simulink model "Guidance"  (R2026a)
settings: Solver=VariableStepAuto
undefined symbols (not defined in the file): ts_uav, waypoints
settings Model: DataDictionary=QuadData.sldd  ModifiedByFormat=The MathWorks, Inc.  Creator=The MathWorks, Inc.  LastModifiedBy=The MathWorks, Inc.

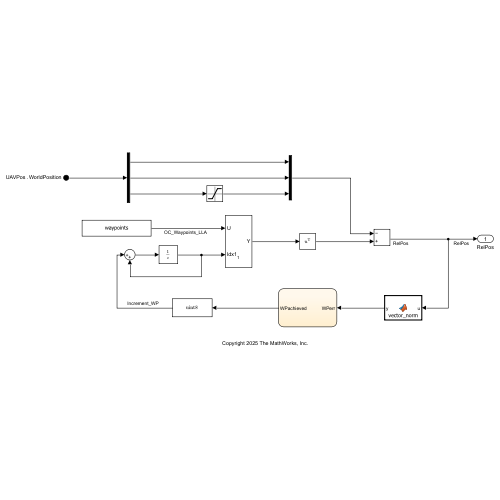
[thumbnail: Simulink's stored preview of the top-level diagram]
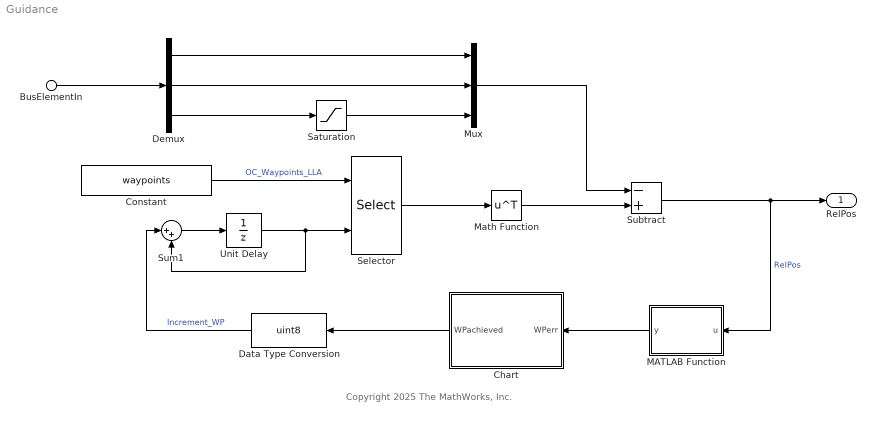
== system Guidance ==
  note: Copyright 2025 The MathWorks, Inc.
  BusElementIn : Inport  PortName=UAVPos  Element=WorldPosition
  Chart : Stateflow chart  TreatAsAtomicUnit=on
  Constant : Constant  Value=waypoints  SampleTime=ts_uav
  Data Type Conversion : DataTypeConversion  OutDataTypeStr=uint8  SaturateOnIntegerOverflow=off  RndMeth=Floor
  Demux : Demux  Outputs=3
  MATLAB Function : MATLAB Function  TreatAsAtomicUnit=on
  Math Function : Math  Operator=transpose
  Mux : Mux  Inputs=3
  Saturation : Saturate  UpperLimit=0.0001  LowerLimit=-inf
  Selector : Selector  NumberOfDimensions=2  InputPortWidth=3  IndexOptions=Starting index (port),Select all  Indices=[1 3],1  OutputSizes=1,1
  Subtract : Sum  Inputs=-+
  Sum1 : Sum  Inputs=|++
  Unit Delay : UnitDelay  InitialCondition=1  SampleTime=-1
  RelPos : Outport
  wires:
  Chart/1(WPachieved) -> Data Type Conversion/1
  Unit Delay/1 -> Sum1/2, Selector/2
  MATLAB Function/1(y) -> Chart/1(WPerr)
  Math Function/1 -> Subtract/2
  Data Type Conversion/1 -> Sum1/1  "Increment_WP"
  Sum1/1 -> Unit Delay/1
  Selector/1 -> Math Function/1
  Subtract/1 -> MATLAB Function/1(u), RelPos/1  "RelPos"
  Constant/1 -> Selector/1  "OC_Waypoints_LLA"
  BusElementIn/1 -> Demux/1
  Demux/3 -> Saturation/1
  Saturation/1 -> Mux/3
  Demux/2 -> Mux/2
  Demux/1 -> Mux/1
  Mux/1 -> Subtract/1

== matlab function Guidance/MATLAB Function ==
  data: u input; y output
function y = vector_norm(u)
    y = norm(u);
end

== stateflow chart Guidance/Chart ==
  state NotNearWP
    en: WPachieved = false;
  state NearWP
    en: count = 0; WPachieved = false;
    du: count = count+ts_uav;
  state WPachieved
    en: WPachieved = true;
  (default) -> NotNearWP
  NotNearWP -> NearWP : [WPerr <= 0.1]
  NearWP -> NotNearWP [order 1] : [WPerr > 0.1]
  WPachieved -> NotNearWP
  NearWP -> WPachieved [order 2] : [count >= 0.75]
  data: WPerr input; count local; WPachieved output; ts_uav parameter
